simulink model "PB2M_001_003_RL"  (R2024a)
settings: Solver=FixedStepDiscrete  StartTime=0.0  StopTime=inf  FixedStep=[global_ST]  RelTol=1e-3
model workspace (MAT data in the model file):
  Var = 0
  imit_action_noise_variance = 0.2
values from neighbouring files (symbols this model uses):
  CGO2_cap = 5000    [SimControl_v3_rl.m]
  global_ST = 1    [SimControl_v3_rl.m]    (also in SimControl_v4.m)
  global_time = [0:1:8784]'    [SimControl_v3_rl.m]    (also in SimControl_v4.m)
undefined symbols (not defined in the file or in its folder): AEL, AMB, ATR, Bttry, CGO2, CHP, COMPR_MIX_E_spec, COMPR_SG_E_spec, DiscIntNeverNeededParam, DIST, DRY, forecast, GASF, Grd, MES, NumEpisodes, NumImitLearning, PV, th, vanilla, WT
libraries: simulink x1, slpidlib x1, rllib x1
(part 2 of 2)

== matlab function PB2M_001_003_RL/ctrl/MATLAB Function ==
  data: El_renew input; CHP output; P_sec input; Battery_lvl input; C_grid input; Battery_in output; Battery_out output; Grid output; P_prim output; curt output; Grd parameter; Bttry parameter; AEL parameter; action input
function [CHP,Battery_in, Battery_out,Grid,P_prim,curt] = manage_power_ex_rl(El_renew, P_sec, Battery_lvl,C_grid,Grd,Bttry,AEL,action)

    CHP = 0;
    Battery_in = 0;
    Battery_out = 0;
    Grid = 0;
    P_prim = El_renew - P_sec;
    curt = 0;

    if P_prim < AEL.Pmin
        action = min(action,0);
        Battery_out = min(action * (P_prim - AEL.Pmin), Battery_lvl - Bttry.min);

        if C_grid <= Grd.cbuy
            Grid = AEL.Pmin - P_prim - Battery_out;
        end
        CHP = AEL.Pmin - P_prim - Battery_out - Grid;  

    elseif AEL.POverload < P_prim
        action = max(0,action);
        Battery_in = min(action * (P_prim - AEL.Pmin), Bttry.Cap - Battery_lvl);
        curt = P_prim - AEL.POverload - Battery_in;

    else
        action = max(0,action);
        Battery_out = 0;
        CHP = 0;
        curt = 0;
        Grid = 0;
        try_Battery_in = action * (P_prim - AEL.Pmin);
        Battery_in = min(try_Battery_in, Bttry.Cap - Battery_lvl);
        P_prim = P_prim - Battery_in;
    end

== matlab function PB2M_001_003_RL/GRID/MATLAB Function1 ==
  data: u input; y output
function y = fcn(u)

if u <= 60
    y = 1;
else
    y = 0;
end

end

== matlab function PB2M_001_003_RL/BM /MATLAB Function ==
  data: mflow_H2 input; module output; mflow_SG input; th parameter; ATR parameter
function module = module_calc(mflow_H2, mflow_SG, th, ATR)
module = module_calc_ex(mflow_H2, mflow_SG, th, ATR);

end
